simulink model "LKS_tcp17"  (R2024b)
settings: Solver=FixedStepAuto  StartTime=0.0  StopTime=2000  FixedStep=0.1  RelTol=1e-3
libraries: simulink x4, simulink_extras x1, instrumentlib x1
settings Model: Creator=28509  LastModifiedBy=ran
settings DataIOCC: SaveFormat=Array  ReturnWorkspaceOutputs=off

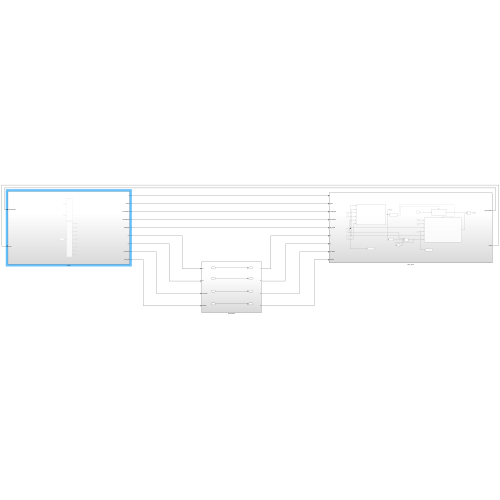
[thumbnail: Simulink's stored preview of the top-level diagram]
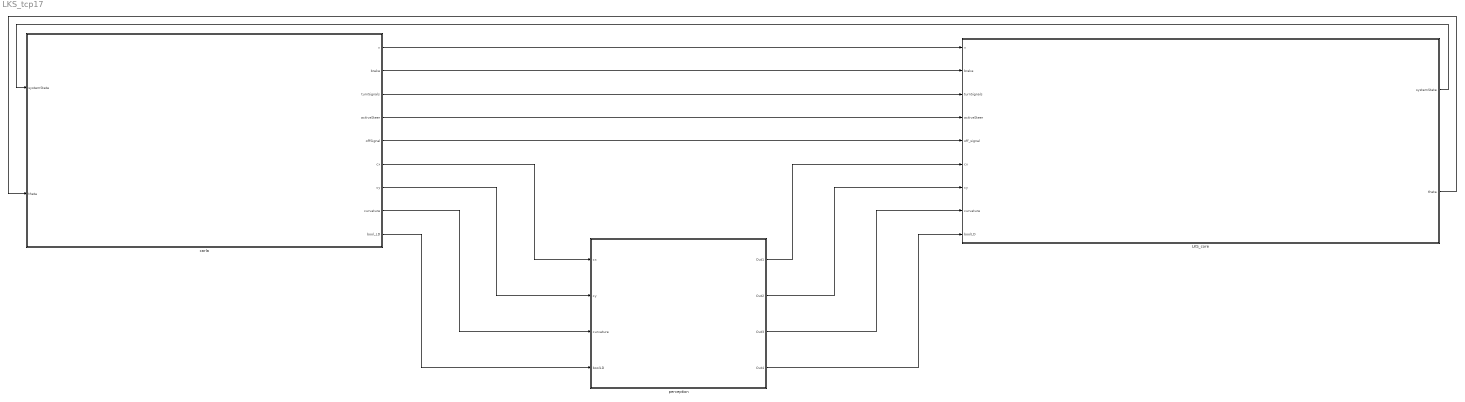
== system LKS_tcp17 ==
  LKS_core : Subsystem
  carla : Subsystem
  perception : Subsystem
  wires:
  perception/1(Out1) -> LKS_core/6(cx)
  perception/2(Out2) -> LKS_core/7(cy)
  carla/8(curvature) -> perception/3(curvature)
  perception/4(Out4) -> LKS_core/9(boolLD)
  LKS_core/2(theta) -> carla/2(theta)
  carla/7(cy) -> perception/2(cy)
  carla/1(v) -> LKS_core/1(v)
  carla/9(bool_LD) -> perception/4(boolLD)
  LKS_core/1(systemState) -> carla/1(systemState)
  perception/3(Out3) -> LKS_core/8(curvature)
  carla/4(activeSteer) -> LKS_core/4(activeSteer)
  carla/2(brake) -> LKS_core/2(brake)
  carla/3(turnSignals) -> LKS_core/3(turnSignals)
  carla/5(offSignal) -> LKS_core/5(off_signal)
  carla/6(cx) -> perception/1(cx)

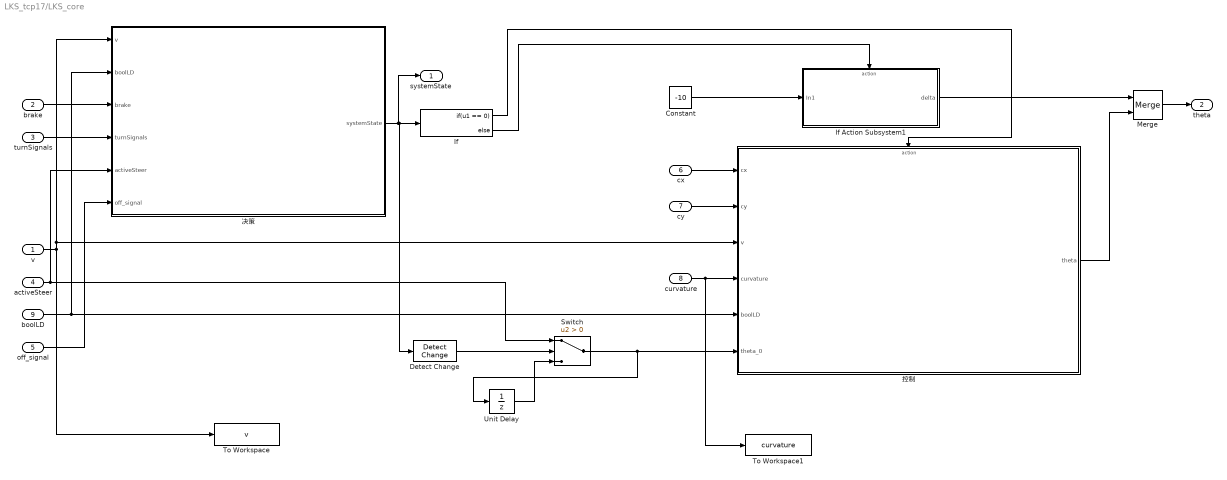
== system LKS_tcp17/LKS_core ==
  v : Inport
  brake : Inport  Port=2
  turnSignals : Inport  Port=3
  activeSteer : Inport  Port=4
  off_signal : Inport  Port=5
  cx : Inport  Port=6
  cy : Inport  Port=7
  curvature : Inport  Port=8
  boolLD : Inport  Port=9
  Constant : Constant  Value=-10
  Detect Change : simulink/Logic and Bit Operations/Detect Change  vinit=0  OutDataTypeStr=uint8
  If : If  IfExpression=u1 == 0
  If Action Subsystem1 : Subsystem  TreatAsAtomicUnit=on
  Merge : Merge
  Switch : Switch  Criteria=u2 > Threshold  SaturateOnIntegerOverflow=off  InputSameDT=off
  To Workspace : ToWorkspace  VariableName=v  SaveFormat=Timeseries  SampleTime=-1
  To Workspace1 : ToWorkspace  VariableName=curvature  SaveFormat=Timeseries  SampleTime=-1
  Unit Delay : UnitDelay  SampleTime=-1  HasFrameUpgradeWarning=on
  决策 : Subsystem
  控制 : Subsystem  TreatAsAtomicUnit=on
  systemState : Outport
  theta : Outport  Port=2
  wires:
  If Action Subsystem1/1(delta) -> Merge/1
  brake/1 -> 决策/3(brake)
  turnSignals/1 -> 决策/4(turnSignals)
  控制/1(theta) -> Merge/2
  off_signal/1 -> 决策/6(off_signal)
  If/2 -> If Action Subsystem1/Action
  Merge/1 -> theta/1
  Constant/1 -> If Action Subsystem1/1(In1)
  boolLD/1 -> 决策/2(boolLD), 控制/5(boolLD)
  If/1 -> 控制/Action
  cx/1 -> 控制/1(cx)
  cy/1 -> 控制/2(cy)
  决策/1(systemState) -> Detect Change/1, If/1, systemState/1
  Detect Change/1 -> Switch/2
  activeSteer/1 -> Switch/1, 决策/5(activeSteer)
  Switch/1 -> Unit Delay/1, 控制/6(theta_0)
  Unit Delay/1 -> Switch/3
  v/1 -> 决策/1(v), 控制/3(v), To Workspace/1
  curvature/1 -> To Workspace1/1, 控制/4(curvature)

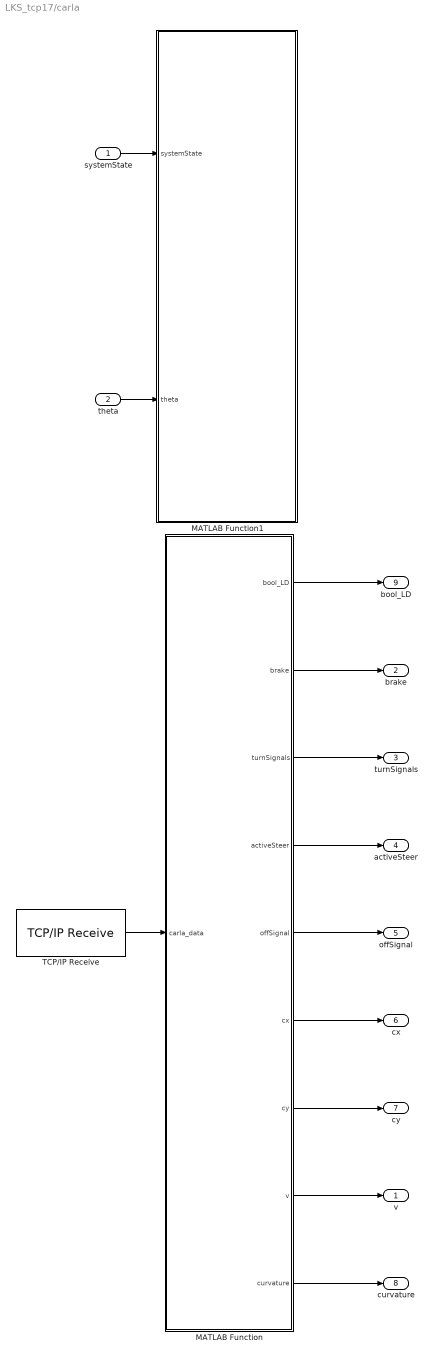
== system LKS_tcp17/carla ==
  systemState : Inport
  theta : Inport  Port=2
  MATLAB Function : MATLAB Function  TreatAsAtomicUnit=on
  MATLAB Function1 : MATLAB Function  TreatAsAtomicUnit=on
  TCP/IP Receive : instrumentlib/TCP//IP Receive  Host=127.0.0.1  Port=25026  DataSize=[1, 186]  DataType=double  ASCIIFormatting=%f  Terminator=LF  CustomTerminator=10  ByteOrder=little-endian  EnableBlockingMode=on  Timeout=5  SampleTime=0.1  SimulateUsing=Interpreted execution
  v : Outport
  brake : Outport  Port=2
  turnSignals : Outport  Port=3
  activeSteer : Outport  Port=4
  offSignal : Outport  Port=5
  cx : Outport  Port=6
  cy : Outport  Port=7
  curvature : Outport  Port=8
  bool_LD : Outport  Port=9
  wires:
  MATLAB Function/9(curvature) -> curvature/1
  MATLAB Function/7(cy) -> cy/1
  MATLAB Function/5(offSignal) -> offSignal/1
  MATLAB Function/8(v) -> v/1
  MATLAB Function/4(activeSteer) -> activeSteer/1
  MATLAB Function/3(turnSignals) -> turnSignals/1
  MATLAB Function/1(bool_LD) -> bool_LD/1
  MATLAB Function/6(cx) -> cx/1
  MATLAB Function/2(brake) -> brake/1
  TCP/IP Receive/1 -> MATLAB Function/1(carla_data)
  theta/1 -> MATLAB Function1/2(theta)
  systemState/1 -> MATLAB Function1/1(systemState)

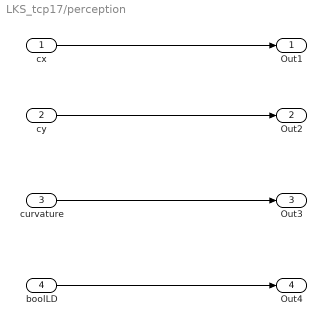
== system LKS_tcp17/perception ==
  cx : Inport
  cy : Inport  Port=2
  curvature : Inport  Port=3
  boolLD : Inport  Port=4
  Out1 : Outport
  Out2 : Outport  Port=2
  Out3 : Outport  Port=3
  Out4 : Outport  Port=4
  wires:
  cx/1 -> Out1/1
  cy/1 -> Out2/1
  curvature/1 -> Out3/1
  boolLD/1 -> Out4/1

== system LKS_tcp17/LKS_core/If Action Subsystem1 ==
  In1 : Inport
  Action Port : ActionPort  ActionPortLabel=else
  delta : Outport
  wires:
  In1/1 -> delta/1

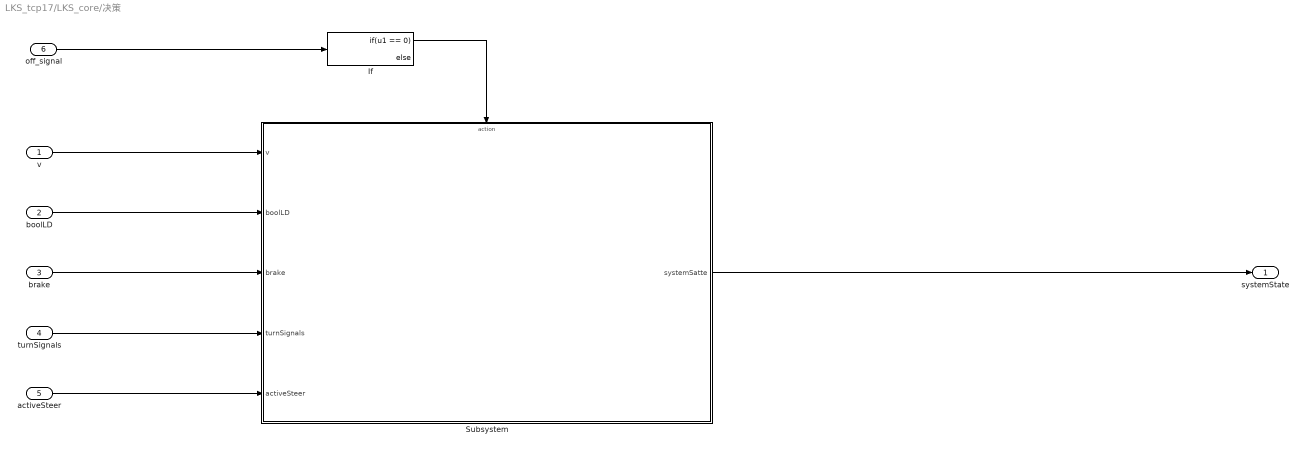
== system LKS_tcp17/LKS_core/决策 ==
  v : Inport
  boolLD : Inport  Port=2
  brake : Inport  Port=3  OutDataTypeStr=double
  turnSignals : Inport  Port=4
  activeSteer : Inport  Port=5
  off_signal : Inport  Port=6
  If : If  IfExpression=u1 == 0
  Subsystem : Subsystem
  systemState : Outport
  wires:
  v/1 -> Subsystem/1(v)
  boolLD/1 -> Subsystem/2(boolLD)
  brake/1 -> Subsystem/3(brake)
  turnSignals/1 -> Subsystem/4(turnSignals)
  activeSteer/1 -> Subsystem/5(activeSteer)
  Subsystem/1(systemSatte) -> systemState/1
  If/1 -> Subsystem/Action
  off_signal/1 -> If/1

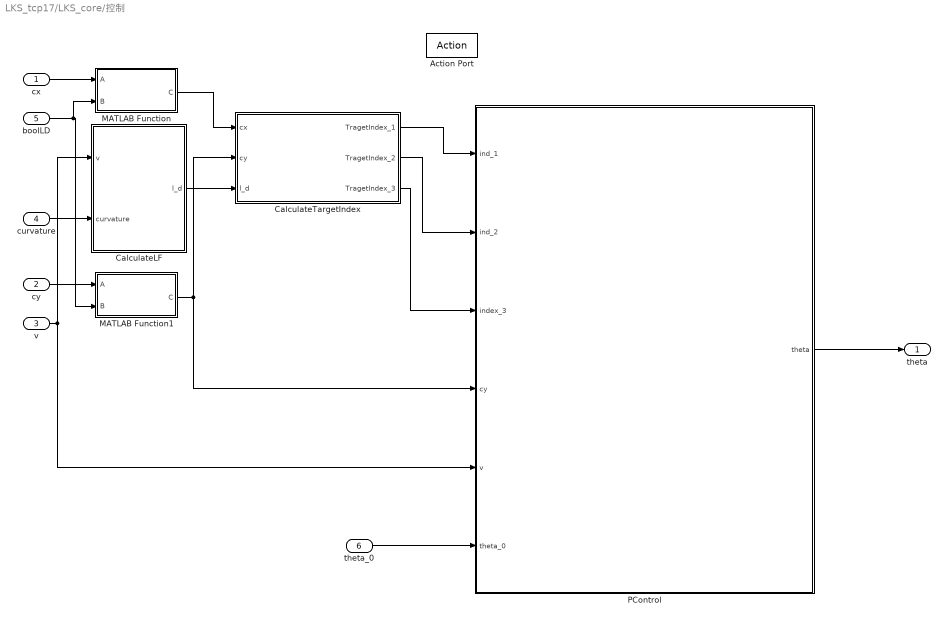
== system LKS_tcp17/LKS_core/控制 ==
  cx : Inport
  cy : Inport  Port=2
  v : Inport  Port=3
  curvature : Inport  Port=4
  boolLD : Inport  Port=5
  theta_0 : Inport  Port=6
  Action Port : ActionPort  ActionPortLabel=if(u1 == 0)
  CalculateLF : Subsystem
  CalculateTargetIndex : Subsystem
  MATLAB Function : MATLAB Function  TreatAsAtomicUnit=on
  MATLAB Function1 : MATLAB Function  TreatAsAtomicUnit=on
  PControl : Subsystem
  theta : Outport  VectorParamsAs1DForOutWhenUnconnected=off
  wires:
  PControl/1(theta) -> theta/1
  cx/1 -> MATLAB Function/1(A)
  boolLD/1 -> MATLAB Function1/2(B), MATLAB Function/2(B)
  v/1 -> CalculateLF/1(v), PControl/5(v)
  cy/1 -> MATLAB Function1/1(A)
  theta_0/1 -> PControl/6(theta_0)
  MATLAB Function/1(C) -> CalculateTargetIndex/1(cx)
  curvature/1 -> CalculateLF/2(curvature)
  MATLAB Function1/1(C) -> CalculateTargetIndex/2(cy), PControl/4(cy)
  CalculateLF/1(l_d) -> CalculateTargetIndex/3(l_d)
  CalculateTargetIndex/2(TragetIndex_2) -> PControl/2(ind_2)
  CalculateTargetIndex/1(TragetIndex_1) -> PControl/1(ind_1)
  CalculateTargetIndex/3(TragetIndex_3) -> PControl/3(index_3)

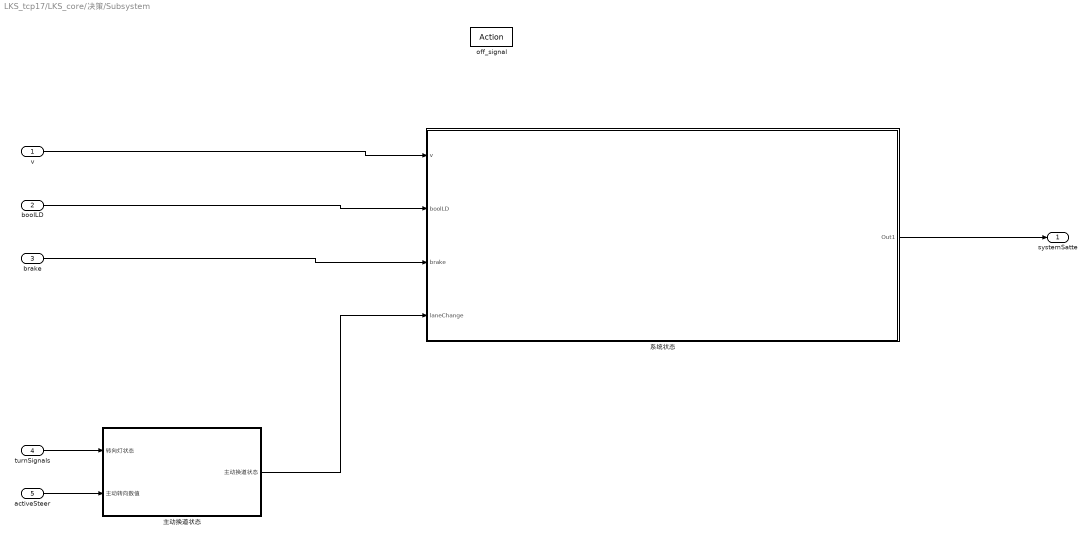
== system LKS_tcp17/LKS_core/决策/Subsystem ==
  v : Inport
  boolLD : Inport  Port=2
  brake : Inport  Port=3  OutDataTypeStr=double
  turnSignals : Inport  Port=4
  activeSteer : Inport  Port=5
  off_signal : ActionPort  ActionPortLabel=if(u1 == 0)
  主动换道状态 : Subsystem
  系统状态 : Subsystem
  systemSatte : Outport
  wires:
  v/1 -> 系统状态/1(v)
  主动换道状态/1(主动换道状态) -> 系统状态/4(laneChange)
  turnSignals/1 -> 主动换道状态/1(转向灯状态)
  activeSteer/1 -> 主动换道状态/2(主动转向数值)
  boolLD/1 -> 系统状态/2(boolLD)
  brake/1 -> 系统状态/3(brake)
  系统状态/1(Out1) -> systemSatte/1

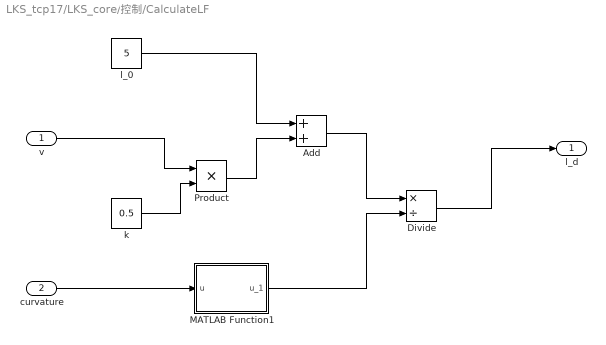
== system LKS_tcp17/LKS_core/控制/CalculateLF ==
  v : Inport
  curvature : Inport  Port=2
  Add : Sum
  Divide : Product  Inputs=*/
  MATLAB Function1 : MATLAB Function  TreatAsAtomicUnit=on
  Product : Product
  k : Constant  Value=0.5
  l_0 : Constant  Value=5
  l_d : Outport
  wires:
  v/1 -> Product/1
  k/1 -> Product/2
  l_0/1 -> Add/1
  Product/1 -> Add/2
  Divide/1 -> l_d/1
  curvature/1 -> MATLAB Function1/1(u)
  Add/1 -> Divide/1
  MATLAB Function1/1(u_1) -> Divide/2

== system LKS_tcp17/LKS_core/控制/CalculateTargetIndex ==
  cx : Inport
  cy : Inport  Port=2
  l_d : Inport  Port=3
  MATLAB Function : MATLAB Function  TreatAsAtomicUnit=on
  TragetIndex_1 : Outport
  TragetIndex_2 : Outport  Port=2
  TragetIndex_3 : Outport  Port=3
  wires:
  cx/1 -> MATLAB Function/1(cx)
  cy/1 -> MATLAB Function/2(cy)
  l_d/1 -> MATLAB Function/3(l_d)
  MATLAB Function/2(index_2) -> TragetIndex_2/1
  MATLAB Function/1(index_1) -> TragetIndex_1/1
  MATLAB Function/3(index_3) -> TragetIndex_3/1

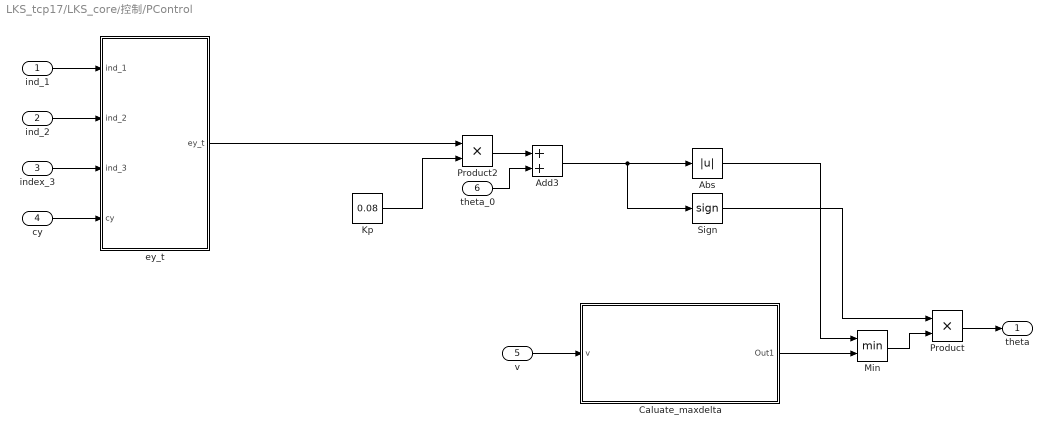
== system LKS_tcp17/LKS_core/控制/PControl ==
  ind_1 : Inport
  ind_2 : Inport  Port=2
  index_3 : Inport  Port=3
  cy : Inport  Port=4
  v : Inport  Port=5
  theta_0 : Inport  Port=6
  Abs : Abs  SaturateOnIntegerOverflow=off
  Add3 : Sum
  Caluate_maxdelta : Subsystem
  Kp : Constant  Value=0.08
  Min : MinMax  Inputs=2
  Product : Product
  Product2 : Product
  Sign : Signum
  ey_t : Subsystem
  theta : Outport  VectorParamsAs1DForOutWhenUnconnected=off
  wires:
  Product/1 -> theta/1
  ind_1/1 -> ey_t/1(ind_1)
  Kp/1 -> Product2/2
  ind_2/1 -> ey_t/2(ind_2)
  theta_0/1 -> Add3/2
  cy/1 -> ey_t/4(cy)
  Abs/1 -> Min/1
  Product2/1 -> Add3/1
  Caluate_maxdelta/1(Out1) -> Min/2
  Add3/1 -> Sign/1, Abs/1
  Min/1 -> Product/2
  v/1 -> Caluate_maxdelta/1(v)
  ey_t/1(ey_t) -> Product2/1
  Sign/1 -> Product/1
  index_3/1 -> ey_t/3(ind_3)

== system LKS_tcp17/LKS_core/决策/Subsystem/主动换道状态 ==
  转向灯状态 : Inport
  主动转向数值 : Inport  Port=2
  Abs : Abs  SaturateOnIntegerOverflow=off
  Add : Sum
  Compare To Constant : simulink/Logic and Bit Operations/Compare To Constant  relop=>=  const=0.05  OutDataTypeStr=boolean
  主动换道状态 : Outport
  wires:
  Compare To Constant/1 -> Add/2
  Add/1 -> 主动换道状态/1
  转向灯状态/1 -> Add/1
  主动转向数值/1 -> Abs/1
  Abs/1 -> Compare To Constant/1

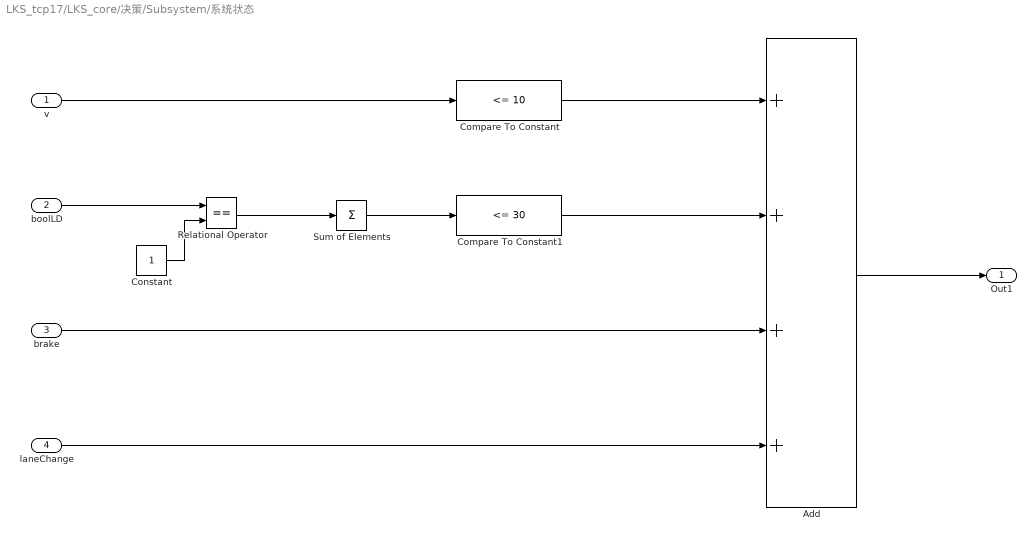
== system LKS_tcp17/LKS_core/决策/Subsystem/系统状态 ==
  v : Inport
  boolLD : Inport  Port=2
  brake : Inport  Port=3
  laneChange : Inport  Port=4
  Add : Sum  Inputs=++++
  Compare To Constant : simulink/Logic and Bit Operations/Compare To Constant  relop=<=  const=10  OutDataTypeStr=boolean
  Compare To Constant1 : simulink/Logic and Bit Operations/Compare To Constant  relop=<=  const=30  OutDataTypeStr=boolean
  Constant : Constant
  Relational Operator : RelationalOperator  Operator===  OutDataTypeStr=boolean  RndMeth=Simplest  InputSameDT=off
  Sum of Elements : Sum  Inputs=+
  Out1 : Outport
  wires:
  boolLD/1 -> Relational Operator/1
  Constant/1 -> Relational Operator/2
  Relational Operator/1 -> Sum of Elements/1
  Add/1 -> Out1/1
  Compare To Constant/1 -> Add/1
  Compare To Constant1/1 -> Add/2
  brake/1 -> Add/3
  laneChange/1 -> Add/4
  v/1 -> Compare To Constant/1
  Sum of Elements/1 -> Compare To Constant1/1

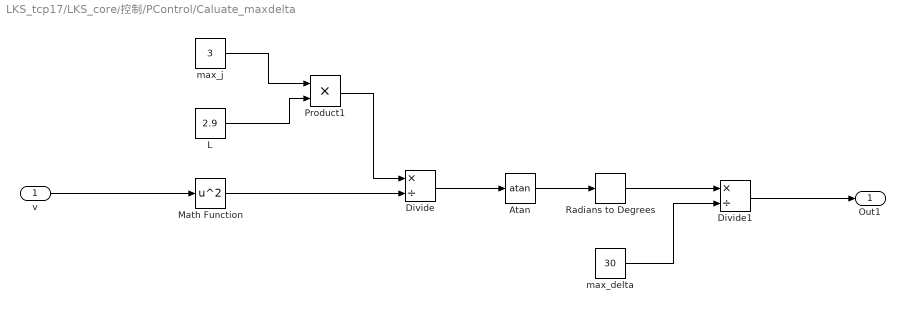
== system LKS_tcp17/LKS_core/控制/PControl/Caluate_maxdelta ==
  v : Inport
  Atan : Trigonometry  Operator=atan
  Divide : Product  Inputs=*/
  Divide1 : Product  Inputs=*/
  L : Constant  Value=2.9
  Math Function : Math  Operator=square
  Product1 : Product
  Radians to Degrees : simulink_extras/Transformations/Radians to Degrees
  max_delta : Constant  Value=30
  max_j : Constant  Value=3
  Out1 : Outport
  wires:
  L/1 -> Product1/2
  v/1 -> Math Function/1
  Divide/1 -> Atan/1
  max_j/1 -> Product1/1
  Divide1/1 -> Out1/1
  Product1/1 -> Divide/1
  max_delta/1 -> Divide1/2
  Math Function/1 -> Divide/2
  Radians to Degrees/1 -> Divide1/1
  Atan/1 -> Radians to Degrees/1

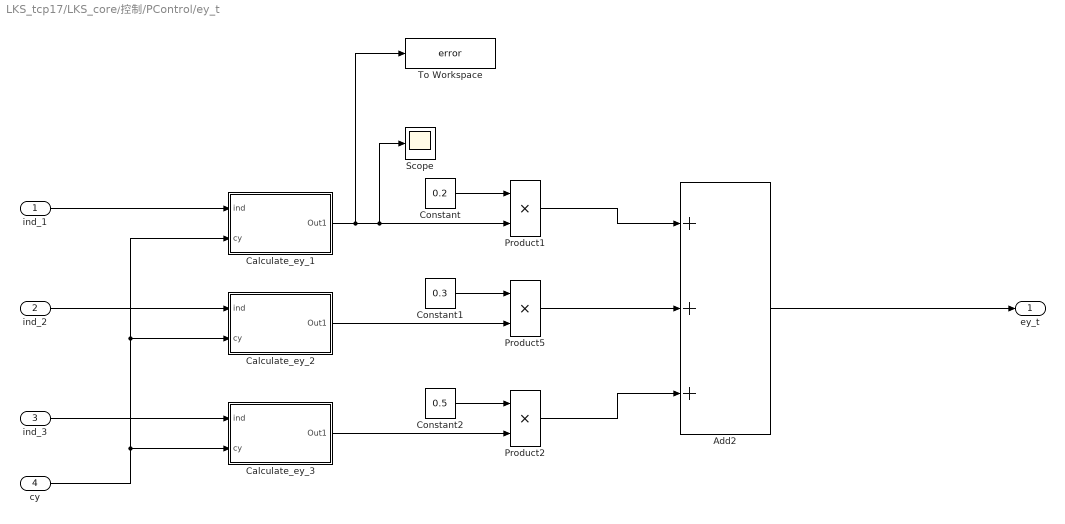
== system LKS_tcp17/LKS_core/控制/PControl/ey_t ==
  ind_1 : Inport
  ind_2 : Inport  Port=2
  ind_3 : Inport  Port=3
  cy : Inport  Port=4
  Add2 : Sum  Inputs=+++
  Calculate_ey_1 : Subsystem
  Calculate_ey_2 : Subsystem
  Calculate_ey_3 : Subsystem
  Constant : Constant  Value=0.2
  Constant1 : Constant  Value=0.3
  Constant2 : Constant  Value=0.5
  Product1 : Product
  Product2 : Product
  Product5 : Product
  Scope : Scope
  To Workspace : ToWorkspace  VariableName=error  SaveFormat=Timeseries  SampleTime=-1
  ey_t : Outport
  wires:
  ind_2/1 -> Calculate_ey_2/1(ind)
  Product1/1 -> Add2/1
  Product5/1 -> Add2/2
  cy/1 -> Calculate_ey_3/2(cy), Calculate_ey_2/2(cy), Calculate_ey_1/2(cy)
  Add2/1 -> ey_t/1
  ind_1/1 -> Calculate_ey_1/1(ind)
  Calculate_ey_2/1(Out1) -> Product5/2
  Calculate_ey_1/1(Out1) -> To Workspace/1, Scope/1, Product1/2
  Constant/1 -> Product1/1
  ind_3/1 -> Calculate_ey_3/1(ind)
  Calculate_ey_3/1(Out1) -> Product2/2
  Constant1/1 -> Product5/1
  Constant2/1 -> Product2/1
  Product2/1 -> Add2/3

== system LKS_tcp17/LKS_core/控制/PControl/ey_t/Calculate_ey_1 ==
  ind : Inport
  cy : Inport  Port=2
  Index Vector2 : MultiPortSwitch  Inputs=1  SaturateOnIntegerOverflow=off  InputSameDT=off
  Out1 : Outport
  wires:
  ind/1 -> Index Vector2/1
  cy/1 -> Index Vector2/2
  Index Vector2/1 -> Out1/1

== system LKS_tcp17/LKS_core/控制/PControl/ey_t/Calculate_ey_2 ==
  ind : Inport
  cy : Inport  Port=2
  Index Vector2 : MultiPortSwitch  Inputs=1  SaturateOnIntegerOverflow=off  InputSameDT=off
  Out1 : Outport
  wires:
  ind/1 -> Index Vector2/1
  cy/1 -> Index Vector2/2
  Index Vector2/1 -> Out1/1

== system LKS_tcp17/LKS_core/控制/PControl/ey_t/Calculate_ey_3 ==
  ind : Inport
  cy : Inport  Port=2
  Index Vector2 : MultiPortSwitch  Inputs=1  SaturateOnIntegerOverflow=off  InputSameDT=off
  Out1 : Outport
  wires:
  ind/1 -> Index Vector2/1
  cy/1 -> Index Vector2/2
  Index Vector2/1 -> Out1/1

== matlab function LKS_tcp17/LKS_core/控制/CalculateTargetIndex/MATLAB Function ==
  data: index_1 output; index_2 output; cx input; cy input; l_d input; index_3 output
function [index_1, index_2, index_3] = calc_target_index(cx, cy, l_d)
    % 初始化索引，防止未找到目标时函数报错
    N = length(cx);
    index_1 = 0; index_2 = 0; index_3 = 0;
    
    % 预计算距离平方，避免在循环内多次计算 sqrt，提升速度
    dist_sq = cx.^2 + cy.^2;
    ld_half_sq = (l_d / 2)^2;
    ld_sq = l_d^2;
    
    % 标志位：记录是否已经找到对应索引
    found1 = false; found2 = false; found3 = false;

    for i = 1:N
        % 逻辑 1: 首个距离 > 0
        if ~found1 && cx(i) > 0
            index_1 = i;
            found1 = true;
        end
        
        % 逻辑 2: 首个距离 > ld/2
        if ~found2 && dist_sq(i) > ld_half_sq
            index_2 = i;
            found2 = true;
        end
        
        % 逻辑 3: 首个距离 > ld
        if ~found3 && dist_sq(i) > ld_sq
            index_3 = i;
            found3 = true;
            break; % 既然 ld 是最大的阈值，找到了就可以直接跳出循环
        end
    end
end

== matlab function LKS_tcp17/carla/MATLAB Function1 ==
  data: systemState input; theta input
function send_simulink_data(systemState,theta)

        host = '127.0.0.1';
        port = 25028;
    
        persistent tcpClient
        if isempty(tcpClient)
            tcpClient = tcpclient(host, port, 'Timeout', 5);
        end
    
    
        data = typecast([double(systemState),double(theta)], 'uint8');
        % Write the byte data to the TCP stream
        write(tcpClient, data);
        %disp("send data successfully data len");
end

== matlab function LKS_tcp17/carla/MATLAB Function ==
  data: bool_LD output; brake output; turnSignals output; activeSteer output; offSignal output; carla_data input; cx output; cy output; v output; curvature output
function [bool_LD,brake,turnSignals,activeSteer,offSignal,cx,cy,v,curvature] = tcp2input(carla_data)
    %disp("carla_data");
    %disp(length(carla_data));
    bool_LD = carla_data(1:60);
    brake = carla_data(61);
    turnSignals = carla_data(62);
    activeSteer = carla_data(63);
    offSignal = carla_data(64);
    %x = carla_data(65);
    %y = carla_data(66);
    v = carla_data(65);
    %disp(v);
    cx = carla_data(66:125);
    cy = carla_data(126:185);
    curvature = carla_data(186);
    
end

== matlab function LKS_tcp17/LKS_core/控制/CalculateLF/MATLAB Function1 ==
  data: u input; u_1 output
function u_1 = fcn(u)
u_1 = 1;
if u >= 0.2
    u_1 = 1.5;
end

== matlab function LKS_tcp17/LKS_core/控制/MATLAB Function ==
  data: A input; C output; B input
function C = filterArray(A, B)
% 输入A和B都是固定大小1x60，输出C最大为1x60，但实际长度取决于B中1的个数
% 将B转换为逻辑索引
mask = logical(B);
% 提取对应元素
temp = A(mask);   % temp是可变长度的向量

% 初始化输出为最大可能长度的向量（用零填充，但实际只使用前一部分）
maxLen = length(A);
C = zeros(1, maxLen);
len = length(temp);
if len > 0
    C(1:len) = temp;
end
end

== matlab function LKS_tcp17/LKS_core/控制/MATLAB Function1 ==
  data: A input; C output; B input
function C = filterArray(A, B)
% 输入A和B都是固定大小1x60，输出C最大为1x60，但实际长度取决于B中1的个数
% 将B转换为逻辑索引
mask = logical(B);
% 提取对应元素
temp = A(mask);   % temp是可变长度的向量

% 初始化输出为最大可能长度的向量（用零填充，但实际只使用前一部分）
maxLen = length(A);
C = zeros(1, maxLen);
len = length(temp);
if len > 0
    C(1:len) = temp;
end
end
